simulink model "chap1_8"  (R2022b)
settings: Solver=ode4  StartTime=0.0  StopTime=1  RelTol=1e-3  EnableMultiTasking=on
settings Model: Creator=Train  LastModifiedBy=Train
settings SolverCC: AlgebraicLoopSolver=TrustRegion
settings DataIOCC: Decimation=100  SaveFormat=Array  SignalLoggingSaveFormat=ModelDataLogs  SaveOutput=off  SaveTime=off  ReturnWorkspaceOutputs=off
settings OptimizationCC: BlockReduction=off  BooleanDataType=off  InitFltsAndDblsToZero=on  LifeSpan=inf
settings DebuggingCC: SaveWithParameterizedLinksMsg=none  UnderspecifiedInitializationDetection=Classic  MergeDetectMultiDrivingBlocksExec=none  SignalResolutionControl=TryResolveAllWithWarning  MultiTaskDSMMsg=warning  MultiTaskCondExecSysMsg=none  FcnCallInpInsideContextMsg=warning  UnconnectedInputMsg=warning  UnconnectedOutputMsg=warning  UnconnectedLineMsg=warning  SFUnexpectedBacktrackingDiag=warning  SFNoUnconditionalDefaultTransitionDiag=warning  SFExecutionAtInitializationDiag=none  SFMachineParentedDataDiag=warning  ArithmeticOperatorsInVariantConditions=warning
settings HardwareCC: ProdBitPerPointer=32  ProdBitPerSizeT=32  ProdBitPerPtrDiffT=32  ProdLargestAtomicFloat=None  ProdIntDivRoundTo=Undefined  ProdEndianess=Unspecified  ProdWordSize=32  ProdHWDeviceType=32-bit Generic  TargetUnknown=on
settings ModelReferenceCC: PropagateSignalLabelsOutOfModel=off
settings CodeAppCC: StateflowObjectComments=on
settings GRTTargetCC: TargetFcnLib=ansi_tfl_tmw.mat  TargetLangStandard=C89/C90 (ANSI)  CombineOutputUpdateFcns=off  GRTInterface=on
settings ConfigComp: CovMetricSettings=dw  CovSaveCumulativeToWorkspaceVar=on  CovSaveSingleToWorkspaceVar=on

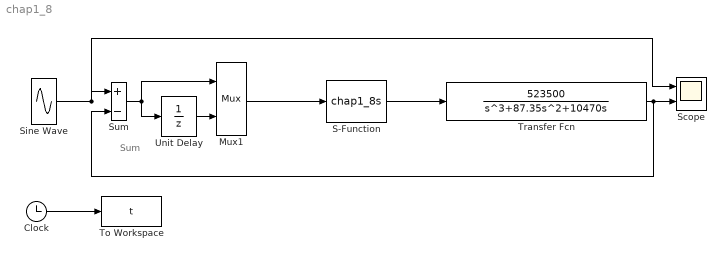
== system chap1_8 ==
  note: Sum
  Clock : Clock
  Mux1 : Mux  Inputs=2
  S-Function : S-Function  FunctionName=chap1_8s  SFunctionDeploymentMode=off  EnableBusSupport=off
  Scope : Scope  NumInputPorts=2
  Sine Wave : Sin  Frequency=1*2*pi  SampleTime=0.001
  Sum : Sum  Inputs=|+-  InputSameDT=on  SaturateOnIntegerOverflow=on  OutDataTypeStr=Inherit: Same as first input
  To Workspace : ToWorkspace  VariableName=t  SampleTime=-1
  Transfer Fcn : TransferFcn  Numerator=[523500]  Denominator=[1 87.35 10470 0]
  Unit Delay : UnitDelay  SampleTime=0.001
  wires:
  Sine Wave/1 -> Scope/1, Sum/1
  Mux1/1 -> S-Function/1
  Unit Delay/1 -> Mux1/2
  Sum/1 -> Mux1/1, Unit Delay/1
  S-Function/1 -> Transfer Fcn/1
  Transfer Fcn/1 -> Scope/2, Sum/2
  Clock/1 -> To Workspace/1
